simulink model "Controle_LQR_Altitude_Foguete_para_Simulink_1"  (R2019a)
settings: Solver=VariableStepAuto  StartTime=0.0  StopTime=5  RelTol=1e-3
undefined symbols (not defined in the file): A, B, K, Ki
settings Model: Creator=Cliente  LastModifiedBy=Cliente

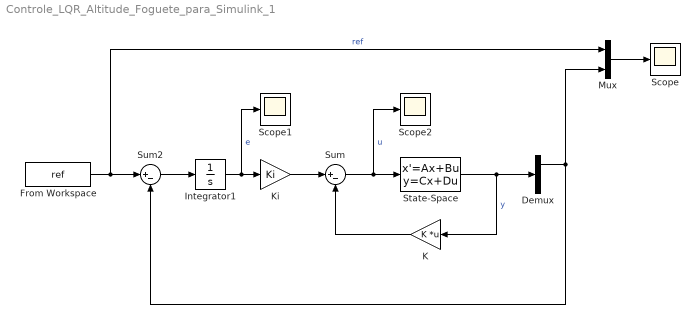
== system Controle_LQR_Altitude_Foguete_para_Simulink_1 ==
  Demux : Demux  Outputs=2
  From Workspace : FromWorkspace  VariableName=ref  SampleTime=0
  Integrator1 : Integrator
  K : Gain  Gain=K  Multiplication=Matrix(K*u) (u vector)
  Ki : Gain  Gain=Ki
  Mux : Mux  Inputs=2
  Scope : Scope
  Scope1 : Scope
  Scope2 : Scope
  State-Space : StateSpace  A=A  B=B  C=eye(2)  D=[0;0]  InitialCondition=[0; 0]
  Sum : Sum  Inputs=|+-
  Sum2 : Sum  Inputs=|+-
  wires:
  K/1 -> Sum/2
  Sum/1 -> Scope2/1, State-Space/1  "u"
  State-Space/1 -> K/1, Demux/1  "y"
  Sum2/1 -> Integrator1/1
  Integrator1/1 -> Scope1/1, Ki/1  "e"
  From Workspace/1 -> Mux/1, Sum2/1  "ref"
  Demux/1 -> Mux/2, Sum2/2
  Mux/1 -> Scope/1
  Ki/1 -> Sum/1
